simulink model "Master_Slave_Model_NOAZ"  (R2019b)
settings: Solver=VariableStepAuto  StartTime=0.0  StopTime=10  RelTol=1e-3
values from neighbouring files (symbols this model uses):
  Be = 5    [parameters.m]
  beta = 2*pi*Fc_h*Ts / (1+2*pi*Fc_h*Ts)    (= 0.0304590279514)    [parameters.m]
  Bh = 2*0.7*sqrt(Kh)    [parameters.m]
  delayCommM2S = 250    [parameters.m]
  delayCommS2M = 250    [parameters.m]
  dt = 0.01    [parameters.m]
  Fc_h = 5    [parameters.m]
  Fh_star = 25    [parameters.m]
  Jh = 0.002    [parameters.m]
  k_m = 19.34    [parameters.m]
  k_s = 19.34    [parameters.m]
  Kc2v_m = 2    [parameters.m]
  Kc2v_s = 2    [parameters.m]
  Kd_h = 0.5    [parameters.m]
  Kd_s = 0.5    [parameters.m]
  Ke = 10    [parameters.m]
  Kh = 25    [parameters.m]
  Kh_max = 50    [parameters.m]
  Kp_h = 1.2    [parameters.m]
  Kp_s = 1    [parameters.m]
  Kt2c_m = 1.182    [parameters.m]
  Kt2c_s = 1.182    [parameters.m]
  lArm_m = 0.1    [parameters.m]
  lArm_s = 0.1    [parameters.m]
  maxCurrent_m = 4.5    [parameters.m]
  maxCurrent_s = 4.5    [parameters.m]
  qe = 0.9    [parameters.m]
  stopTime = str2double(stopTime)    [parameters.m]
  tau_s = 1.217    [parameters.m]
  Ts = 0.001    [parameters.m]
  Variance = 0.0001    [parameters.m]
libraries: simulink_extras x16, dspsigops x16, dspsrcs4 x1
settings Model: Creator=Mirko  LastModifiedBy=Mirko

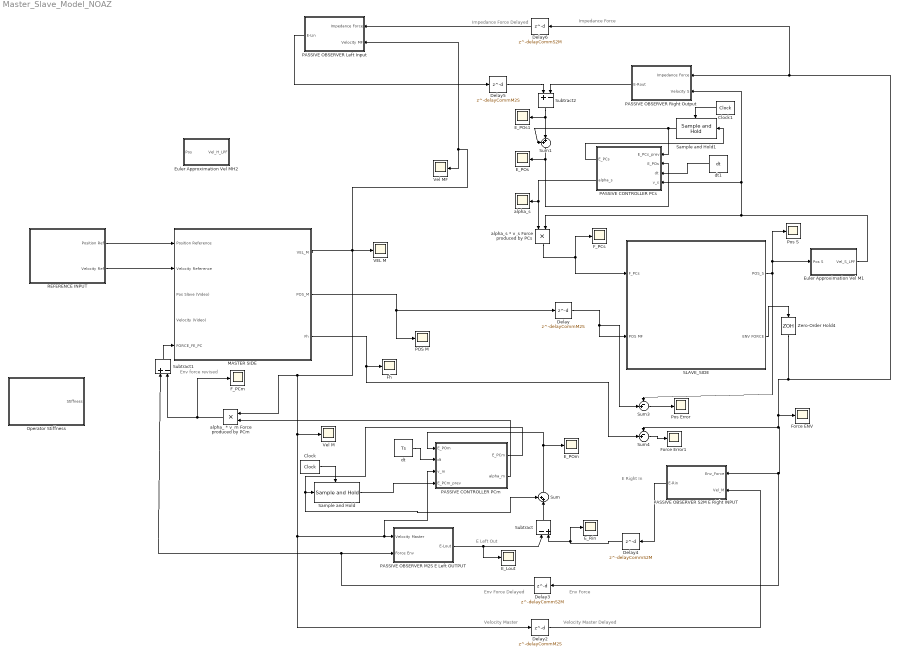
== system Master_Slave_Model_NOAZ ==
  note: Impedance Force Delayed
  note: Impedance Force
  note: Env force revised
  note: E Right In
  note: E Left Out
  note: Env Force Delayed
  note: Env Force
  note: Velocity Master
  note: Velocity Master Delayed
  Clock : simulink_extras/Flip Flops/Clock  period=Ts
  Clock1 : simulink_extras/Flip Flops/Clock  period=Ts
  Delay : Delay  DelayLength=delayCommM2S  InitialCondition=0  SampleTime=Ts
  Delay2 : Delay  DelayLength=delayCommM2S  InitialCondition=0  SampleTime=Ts
  Delay3 : Delay  DelayLength=delayCommS2M  InitialCondition=0  SampleTime=Ts
  Delay4 : Delay  DelayLength=delayCommS2M  InitialCondition=0
  Delay5 : Delay  DelayLength=delayCommM2S  InitialCondition=0  SampleTime=Ts
  Delay6 : Delay  DelayLength=delayCommS2M  InitialCondition=0  SampleTime=Ts
  E_Lout : Scope
  E_POm : Scope
  E_POs : Scope
  E_POs1 : Scope
  E_Rin : Scope
  Euler Approximation Vel M1 : Subsystem
  Euler Approximation Vel MH2 : Subsystem
  F_PCm : Scope
  F_PCs : Scope
  "Fh " : Scope
  Force ENV : Scope
  Force Error1 : Scope
  MASTER SIDE : Subsystem
  Operator Stiffness : Subsystem
  PASSIVE CONTROLLER PCm : MATLAB Function  TreatAsAtomicUnit=on
  PASSIVE CONTROLLER PCs : MATLAB Function  TreatAsAtomicUnit=on
  PASSIVE OBSERVER Left Input : Subsystem
  PASSIVE OBSERVER Right Output : Subsystem
  PASSIVE OBSERVER M2S E Left OUTPUT : Subsystem
  PASSIVE OBSERVER S2M E Right INPUT : Subsystem
  "POS M " : Scope
  Pos Error : Scope
  Pos S : Scope
  REFERENCE INPUT : Subsystem
  "SLAVE_SIDE " : Subsystem
  Sample and Hold : dspsigops/Sample and Hold  trig=Rising edge  initCond=0  latchinput=on
  Sample and Hold1 : dspsigops/Sample and Hold  trig=Rising edge  initCond=0  latchinput=on
  Subtract : Sum  Inputs=-|+
  Subtract1 : Sum  Inputs=+|-
  Subtract2 : Sum  Inputs=+|-
  Sum : Sum  Inputs=++|
  Sum1 : Sum  Inputs=++|
  Sum3 : Sum  Inputs=-+|
  Sum4 : Sum  Inputs=-+|
  VEL M : Scope
  "Vel M " : Scope
  Vel MF : Scope
  Zero-Order Hold4 : ZeroOrderHold  SampleTime=Ts
  alpha_ * v_m Force produced by PCm : Product
  alpha_s : Scope
  alpha_s * v_s Force produced by PCs : Product
  dt : Constant  Value=Ts
  dt1 : Constant  Value=dt
  wires:
  Delay3/1 -> PASSIVE OBSERVER M2S E Left OUTPUT/2(Force Env), Subtract1/1
  Delay2/1 -> PASSIVE OBSERVER S2M E Right INPUT/2("Vel_M ")
  PASSIVE OBSERVER M2S E Left OUTPUT/1(E-Lout) -> E_Lout/1, Subtract/1
  Subtract/1 -> Sum/2
  dt/1 -> PASSIVE CONTROLLER PCm/2(dt)
  PASSIVE CONTROLLER PCm/1(E_PCm) -> Sum/1, Sample and Hold/1
  Sum/1 -> E_POm/1, PASSIVE CONTROLLER PCm/1(E_POm)
  PASSIVE CONTROLLER PCm/2(alpha_m) -> alpha_ * v_m Force produced by PCm/2
  alpha_ * v_m Force produced by PCm/1 -> Subtract1/2, F_PCm/1
  Delay6/1 -> PASSIVE OBSERVER Left Input/1(Impedance Force)
  PASSIVE OBSERVER S2M E Right INPUT/1(E-Rin) -> Delay4/1
  Delay4/1 -> E_Rin/1, Subtract/2
  Euler Approximation Vel M1/1("Vel_S_LPF ") -> alpha_s * v_s Force produced by PCs/2, PASSIVE OBSERVER Right Output/2(Velocity S), PASSIVE CONTROLLER PCs/4(v_s)
  PASSIVE OBSERVER Left Input/1(E-Lin) -> Delay5/1
  Delay5/1 -> Subtract2/1
  PASSIVE OBSERVER Right Output/1(E-Rout) -> Subtract2/2
  dt1/1 -> PASSIVE CONTROLLER PCs/3(dt)
  Subtract2/1 -> E_POs1/1, Sum1/2
  PASSIVE CONTROLLER PCs/1(E_PCs) -> Sample and Hold1/1
  Sum1/1 -> E_POs/1, PASSIVE CONTROLLER PCs/2(E_POs)
  PASSIVE CONTROLLER PCs/2(alpha_s) -> alpha_s/1, alpha_s * v_s Force produced by PCs/1
  alpha_s * v_s Force produced by PCs/1 -> F_PCs/1, "SLAVE_SIDE "/1(F_PCs)
  Subtract1/1 -> MASTER SIDE/5("FORCE_FE_PC ")
  REFERENCE INPUT/1("Position Ref ") -> MASTER SIDE/1(Position Reference)
  Sum3/1 -> Pos Error/1
  Sum4/1 -> Force Error1/1
  MASTER SIDE/1(VEL_M) -> VEL M/1, PASSIVE OBSERVER Left Input/2(Velocity MF), Vel MF/1, alpha_ * v_m Force produced by PCm/1, "Vel M "/1, PASSIVE CONTROLLER PCm/3(v_m), PASSIVE OBSERVER M2S E Left OUTPUT/1(Velocity Master), Delay2/1
  Delay/1 -> Sum3/2, "SLAVE_SIDE "/2(POS MF)
  MASTER SIDE/3(Fh) -> Sum4/2, "Fh "/1
  "SLAVE_SIDE "/2(ENV FORCE) -> Zero-Order Hold4/1
  Zero-Order Hold4/1 -> Force ENV/1, PASSIVE OBSERVER S2M E Right INPUT/1(Env_Force), Delay3/1, Sum4/1, Delay6/1, PASSIVE OBSERVER Right Output/1(Impedance Force)
  MASTER SIDE/2(POS_M) -> "POS M "/1, Delay/1
  "SLAVE_SIDE "/1(POS_S) -> Euler Approximation Vel M1/1(Pos S), Pos S/1, Sum3/1
  Sample and Hold/1 -> PASSIVE CONTROLLER PCm/4(E_PCm_prev)
  Clock/1 -> Sample and Hold/Trigger
  Sample and Hold1/1 -> PASSIVE CONTROLLER PCs/1(E_PCs_prev), Sum1/1
  Clock1/1 -> Sample and Hold1/Trigger
  REFERENCE INPUT/2("Velocity Ref ") -> MASTER SIDE/2(Velocity Reference)

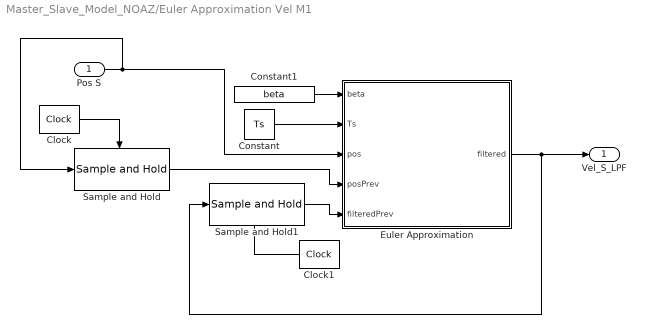
== system Master_Slave_Model_NOAZ/Euler Approximation Vel M1 ==
  Pos S : Inport
  Clock : simulink_extras/Flip Flops/Clock  period=Ts
  Clock1 : simulink_extras/Flip Flops/Clock  period=Ts
  Constant : Constant  Value=Ts
  Constant1 : Constant  Value=beta
  "Euler Approximation " : MATLAB Function  TreatAsAtomicUnit=on
  Sample and Hold : dspsigops/Sample and Hold  trig=Rising edge  initCond=0  latchinput=on
  Sample and Hold1 : dspsigops/Sample and Hold  trig=Rising edge  initCond=0  latchinput=on
  "Vel_S_LPF " : Outport
  wires:
  Pos S/1 -> Sample and Hold/1, "Euler Approximation "/3(pos)
  Constant/1 -> "Euler Approximation "/2(Ts)
  Sample and Hold/1 -> "Euler Approximation "/4(posPrev)
  Clock/1 -> Sample and Hold/Trigger
  Sample and Hold1/1 -> "Euler Approximation "/5(filteredPrev)
  "Euler Approximation "/1(filtered) -> "Vel_S_LPF "/1, Sample and Hold1/1
  Clock1/1 -> Sample and Hold1/Trigger
  Constant1/1 -> "Euler Approximation "/1(beta)

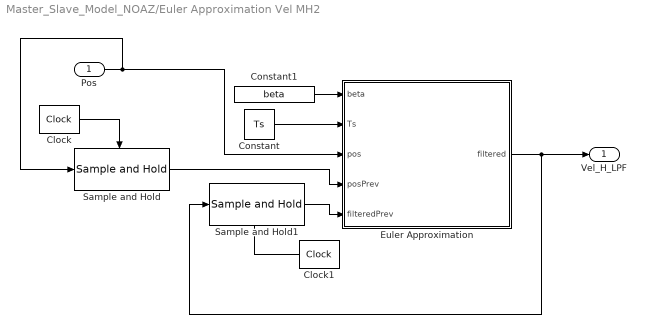
== system Master_Slave_Model_NOAZ/Euler Approximation Vel MH2 ==
  Pos : Inport
  Clock : simulink_extras/Flip Flops/Clock  period=Ts
  Clock1 : simulink_extras/Flip Flops/Clock  period=Ts
  Constant : Constant  Value=Ts
  Constant1 : Constant  Value=beta
  "Euler Approximation " : MATLAB Function  TreatAsAtomicUnit=on
  Sample and Hold : dspsigops/Sample and Hold  trig=Rising edge  initCond=0  latchinput=on
  Sample and Hold1 : dspsigops/Sample and Hold  trig=Rising edge  initCond=0  latchinput=on
  "Vel_H_LPF " : Outport
  wires:
  Pos/1 -> Sample and Hold/1, "Euler Approximation "/3(pos)
  Constant/1 -> "Euler Approximation "/2(Ts)
  Sample and Hold/1 -> "Euler Approximation "/4(posPrev)
  Clock/1 -> Sample and Hold/Trigger
  Sample and Hold1/1 -> "Euler Approximation "/5(filteredPrev)
  "Euler Approximation "/1(filtered) -> "Vel_H_LPF "/1, Sample and Hold1/1
  Clock1/1 -> Sample and Hold1/Trigger
  Constant1/1 -> "Euler Approximation "/1(beta)

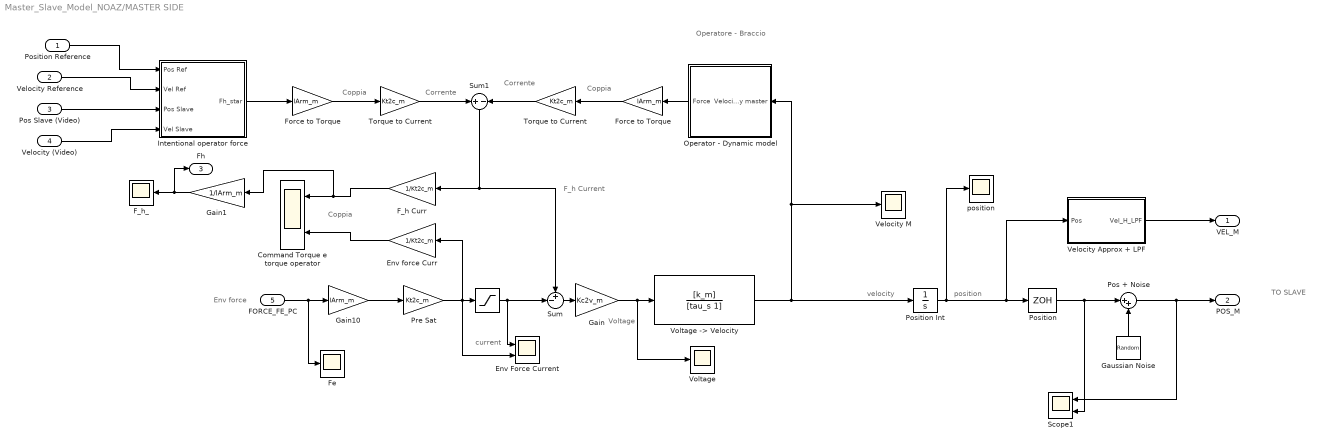
== system Master_Slave_Model_NOAZ/MASTER SIDE ==
  note: Env force
  note: F_h Current
  note: Coppia
  note: Corrente
  note: Coppia
  note: Corrente
  note: Coppia
  note: Operatore - Braccio
  note: current
  note: Voltage
  note: position
  note: velocity
  note: TO SLAVE
  Position Reference : Inport
  Velocity Reference : Inport  Port=2
  Pos Slave (Video) : Inport  Port=3
  Velocity (Video) : Inport  Port=4
  "FORCE_FE_PC " : Inport  Port=5
  " " : Saturate  UpperLimit=maxCurrent_m  LowerLimit=-maxCurrent_m
  "Command Torque e torque operator " : Scope  NumInputPorts=2
  Env Force Current : Scope  NumInputPorts=2
  Env force Curr : Gain  Gain=1/Kt2c_m
  F_h Curr : Gain  Gain=1/Kt2c_m
  "F_h_ " : Scope
  Fe : Scope
  Force to Torque : Gain  Gain=lArm_m
  "Force to Torque " : Gain  Gain=lArm_m
  Gain : Gain  Gain=Kc2v_m
  Gain1 : Gain  Gain=1/lArm_m
  Gain10 : Gain  Gain=lArm_m
  "Gaussian Noise " : RandomNumber  Variance=Variance  SampleTime=Ts
  Intentional operator force : Subsystem
  Operator - Dynamic model : Subsystem
  Pos + Noise : Sum  Inputs=|++
  Position : ZeroOrderHold  SampleTime=Ts
  "Position Int " : Integrator
  Pre Sat : Gain  Gain=Kt2c_m
  Scope1 : Scope  NumInputPorts=2
  Sum : Sum  Inputs=+-|
  Sum1 : Sum  Inputs=+-
  Torque to Current : Gain  Gain=Kt2c_m
  "Torque to Current " : Gain  Gain=Kt2c_m
  "Velocity Approx + LPF " : Subsystem
  Velocity M : Scope
  Voltage : Scope
  "Voltage -> Velocity" : TransferFcn  Numerator=[k_m]  Denominator=[tau_s 1]
  position : Scope
  VEL_M : Outport
  POS_M : Outport  Port=2
  Fh : Outport  Port=3
  wires:
  Pre Sat/1 -> Env Force Current/2, Env force Curr/1, " "/1
  "Position Int "/1 -> "Velocity Approx + LPF "/1(Pos), Position/1, position/1
  "Voltage -> Velocity"/1 -> Velocity M/1, Operator - Dynamic model/1("Velocity master "), "Position Int "/1
  Sum1/1 -> Sum/1, F_h Curr/1
  "Force to Torque "/1 -> Torque to Current/1
  F_h Curr/1 -> Gain1/1, "Command Torque e torque operator "/1
  Force to Torque/1 -> "Torque to Current "/1
  "Torque to Current "/1 -> Sum1/2
  Env force Curr/1 -> "Command Torque e torque operator "/2
  Torque to Current/1 -> Sum1/1
  Position Reference/1 -> Intentional operator force/1(Pos Ref)
  Gain/1 -> Voltage/1, "Voltage -> Velocity"/1
  Sum/1 -> Gain/1
  "FORCE_FE_PC "/1 -> Fe/1, Gain10/1
  Gain10/1 -> Pre Sat/1
  Operator - Dynamic model/1(Force) -> Force to Torque/1
  " "/1 -> Sum/2, Env Force Current/1
  Gain1/1 -> Fh/1, "F_h_ "/1
  "Gaussian Noise "/1 -> Pos + Noise/2
  Pos + Noise/1 -> Scope1/1, POS_M/1
  Position/1 -> Scope1/2, Pos + Noise/1
  "Velocity Approx + LPF "/1("Vel_H_LPF ") -> VEL_M/1
  Velocity Reference/1 -> Intentional operator force/2(Vel Ref)
  Intentional operator force/1("Fh_star ") -> "Force to Torque "/1
  Pos Slave (Video)/1 -> Intentional operator force/3(Pos Slave)
  Velocity (Video)/1 -> Intentional operator force/4(Vel Slave)

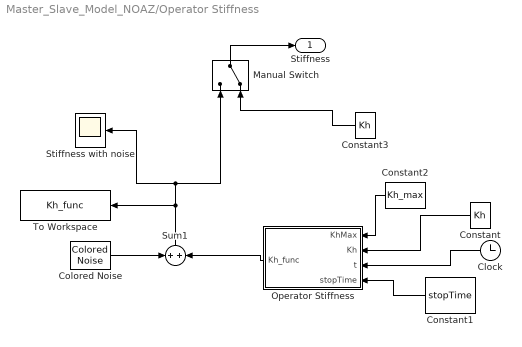
== system Master_Slave_Model_NOAZ/Operator Stiffness ==
  Clock : Clock
  Colored Noise : dspsrcs4/Colored Noise  Color=white  InverseFrequencyPower=1  BoundedOutput=off  NumChannels=1  OutputDataType=double  SamplesPerFrame=1  SampleTime=0.01  RandomStream=mt19937ar with seed  Seed=67  SimulateUsing=Interpreted execution
      settings: SourceProductName=DSP System Toolbox  SourceProductBaseCode=DS
  Constant : Constant  Value=Kh
  Constant1 : Constant  Value=stopTime
  Constant2 : Constant  Value=Kh_max
  Constant3 : Constant  Value=Kh
  Manual Switch : ManualSwitch  CurrentSetting=0
  "Operator Stiffness " : MATLAB Function  TreatAsAtomicUnit=on
  Stiffness with noise : Scope
  Sum1 : Sum
  To Workspace : ToWorkspace  VariableName=Kh_func  SaveFormat=Structure With Time  SampleTime=-1
      settings: Save2DSignal=2-D array (concatenate along first dimension)
  Stiffness : Outport
  wires:
  Constant3/1 -> Manual Switch/2
  Sum1/1 -> To Workspace/1, Manual Switch/1, Stiffness with noise/1
  Constant2/1 -> "Operator Stiffness "/1(KhMax)
  "Operator Stiffness "/1(Kh_func) -> Sum1/2
  Clock/1 -> "Operator Stiffness "/3(t)
  Colored Noise/1 -> Sum1/1
  Constant/1 -> "Operator Stiffness "/2(Kh)
  Constant1/1 -> "Operator Stiffness "/4(stopTime)
  Manual Switch/1 -> Stiffness/1

== system Master_Slave_Model_NOAZ/PASSIVE OBSERVER Left Input ==
  Impedance Force : Inport
  Velocity MF : Inport  Port=2
  Add : Sum
  Clock : simulink_extras/Flip Flops/Clock  period=Ts
  Product : Product
  Sample and Hold : dspsigops/Sample and Hold  trig=Rising edge  initCond=0  latchinput=on
  E-Lin : Outport
  wires:
  Velocity MF/1 -> Product/1
  Impedance Force/1 -> Product/2
  Product/1 -> Add/2
  Sample and Hold/1 -> Add/1
  Add/1 -> Sample and Hold/1, E-Lin/1
  Clock/1 -> Sample and Hold/Trigger

== system Master_Slave_Model_NOAZ/PASSIVE OBSERVER Right Output ==
  Impedance Force : Inport
  Velocity S : Inport  Port=2
  Add : Sum
  Clock : simulink_extras/Flip Flops/Clock  period=Ts
  Product : Product
  Sample and Hold : dspsigops/Sample and Hold  trig=Rising edge  initCond=0  latchinput=on
  E-Rout : Outport
  wires:
  Velocity S/1 -> Product/1
  Impedance Force/1 -> Product/2
  Product/1 -> Add/2
  Sample and Hold/1 -> Add/1
  Add/1 -> Sample and Hold/1, E-Rout/1
  Clock/1 -> Sample and Hold/Trigger

== system Master_Slave_Model_NOAZ/PASSIVE OBSERVER M2S E Left OUTPUT ==
  Velocity Master : Inport
  Force Env : Inport  Port=2
  Add : Sum
  Clock : simulink_extras/Flip Flops/Clock  period=Ts
  Product : Product
  Sample and Hold : dspsigops/Sample and Hold  trig=Rising edge  initCond=0  latchinput=on
  E-Lout : Outport
  wires:
  Velocity Master/1 -> Product/1
  Force Env/1 -> Product/2
  Product/1 -> Add/2
  Sample and Hold/1 -> Add/1
  Add/1 -> Sample and Hold/1, E-Lout/1
  Clock/1 -> Sample and Hold/Trigger

== system Master_Slave_Model_NOAZ/PASSIVE OBSERVER S2M E Right INPUT ==
  Env_Force : Inport
  "Vel_M " : Inport  Port=2
  Add : Sum
  Clock : simulink_extras/Flip Flops/Clock  period=Ts
  Product : Product
  Sample and Hold : dspsigops/Sample and Hold  trig=Rising edge  initCond=0  latchinput=on
  E-Rin : Outport
  wires:
  Env_Force/1 -> Product/1
  "Vel_M "/1 -> Product/2
  Product/1 -> Add/2
  Add/1 -> Sample and Hold/1, E-Rin/1
  Sample and Hold/1 -> Add/1
  Clock/1 -> Sample and Hold/Trigger

== system Master_Slave_Model_NOAZ/REFERENCE INPUT ==
  Derivative : Derivative
  Manual Switch : ManualSwitch  CurrentSetting=0
  Sine Wave : Sin  Amplitude=Fh_star  SampleTime=0
  Step : Step  After=Fh_star  SampleTime=0
  Transfer Fcn : TransferFcn  Numerator=[2*pi*Fc_h]  Denominator=[1 2*pi*Fc_h]
  "Position Ref " : Outport
  "Velocity Ref " : Outport  Port=2
  wires:
  Sine Wave/1 -> Manual Switch/1
  Step/1 -> Transfer Fcn/1
  Transfer Fcn/1 -> Manual Switch/2
  Manual Switch/1 -> Derivative/1, "Position Ref "/1
  Derivative/1 -> "Velocity Ref "/1

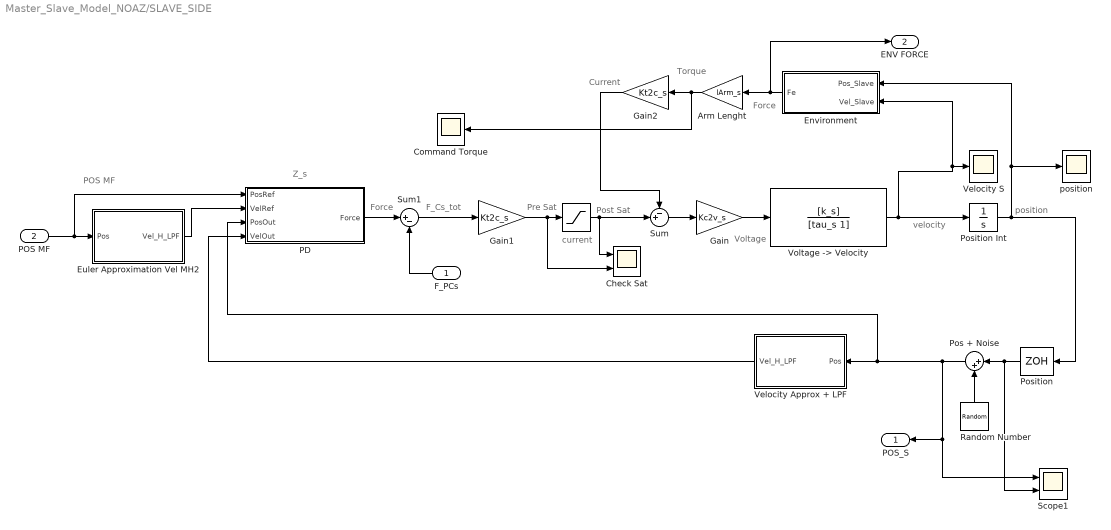
== system Master_Slave_Model_NOAZ/SLAVE_SIDE  ==
  note: Post Sat
  note: Pre Sat
  note: POS MF
  note: current
  note: Force
  note: velocity
  note: position
  note: Current
  note: Voltage
  note: Torque
  note: Z_s
  note: Force
  note: F_Cs_tot
  F_PCs : Inport
  POS MF : Inport  Port=2
  " " : Saturate  UpperLimit=maxCurrent_s  LowerLimit=-maxCurrent_s
  Arm Lenght : Gain  Gain=lArm_s
  Check Sat : Scope  NumInputPorts=2
  Command Torque : Scope
  "Environment " : Subsystem
  Euler Approximation Vel MH2 : Subsystem
  Gain : Gain  Gain=Kc2v_s
  Gain1 : Gain  Gain=Kt2c_s
  Gain2 : Gain  Gain=Kt2c_s
  PD : Subsystem
  Pos + Noise : Sum  Inputs=|++
  Position : ZeroOrderHold  SampleTime=Ts
  Position Int : Integrator
  Random Number : RandomNumber  Variance=Variance  SampleTime=Ts
  Scope1 : Scope  NumInputPorts=2
  Sum : Sum  Inputs=-+|
  Sum1 : Sum  Inputs=|+-
  "Velocity Approx + LPF " : Subsystem
  Velocity S : Scope
  "Voltage -> Velocity " : TransferFcn  Numerator=[k_s]  Denominator=[tau_s 1]
  position : Scope
  POS_S : Outport
  ENV FORCE : Outport  Port=2
  wires:
  PD/1(Force) -> Sum1/1
  Gain1/1 -> Check Sat/2, " "/1
  Gain2/1 -> Sum/1
  "Environment "/1(Fe) -> ENV FORCE/1, Arm Lenght/1
  "Voltage -> Velocity "/1 -> Position Int/1, Velocity S/1, "Environment "/2("Vel_Slave ")
  Sum/1 -> Gain/1
  Gain/1 -> "Voltage -> Velocity "/1
  Sum1/1 -> Gain1/1
  " "/1 -> Check Sat/1, Sum/2
  Arm Lenght/1 -> Command Torque/1, Gain2/1
  F_PCs/1 -> Sum1/2
  Euler Approximation Vel MH2/1("Vel_H_LPF ") -> PD/2(VelRef)
  POS MF/1 -> PD/1(PosRef), Euler Approximation Vel MH2/1(Pos)
  Random Number/1 -> Pos + Noise/2
  Pos + Noise/1 -> PD/3(PosOut), "Velocity Approx + LPF "/1(Pos), POS_S/1, Scope1/1
  Position/1 -> Scope1/2, Pos + Noise/1
  Position Int/1 -> Position/1, position/1, "Environment "/1(Pos_Slave)
  "Velocity Approx + LPF "/1("Vel_H_LPF ") -> PD/4(VelOut)

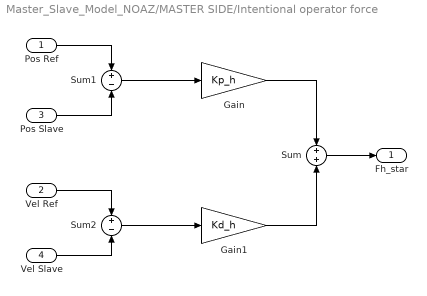
== system Master_Slave_Model_NOAZ/MASTER SIDE/Intentional operator force ==
  Pos Ref : Inport
  Vel Ref : Inport  Port=2
  Pos Slave : Inport  Port=3
  Vel Slave : Inport  Port=4
  Gain : Gain  Gain=Kp_h
  Gain1 : Gain  Gain=Kd_h
  Sum : Sum
  Sum1 : Sum  Inputs=+-
  Sum2 : Sum  Inputs=+-
  "Fh_star " : Outport
  wires:
  Sum/1 -> "Fh_star "/1
  Pos Ref/1 -> Sum1/1
  Pos Slave/1 -> Sum1/2
  Vel Ref/1 -> Sum2/1
  Vel Slave/1 -> Sum2/2
  Sum1/1 -> Gain/1
  Sum2/1 -> Gain1/1
  Gain1/1 -> Sum/2
  Gain/1 -> Sum/1

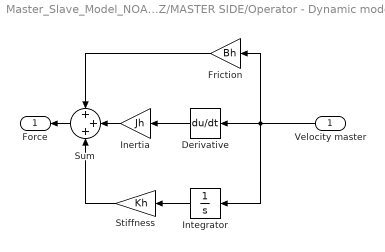
== system Master_Slave_Model_NOAZ/MASTER SIDE/Operator - Dynamic model ==
  "Velocity master " : Inport
  Derivative : Derivative  CoefficientInTFapproximation=0.01
  Friction : Gain  Gain=Bh
  Inertia : Gain  Gain=Jh
  Integrator : Integrator
  "Stiffness " : Gain  Gain=Kh
  Sum : Sum  Inputs=+++
  Force : Outport
  wires:
  "Velocity master "/1 -> Friction/1, Integrator/1, Derivative/1
  Derivative/1 -> Inertia/1
  Inertia/1 -> Sum/2
  Friction/1 -> Sum/1
  Sum/1 -> Force/1
  Integrator/1 -> "Stiffness "/1
  "Stiffness "/1 -> Sum/3

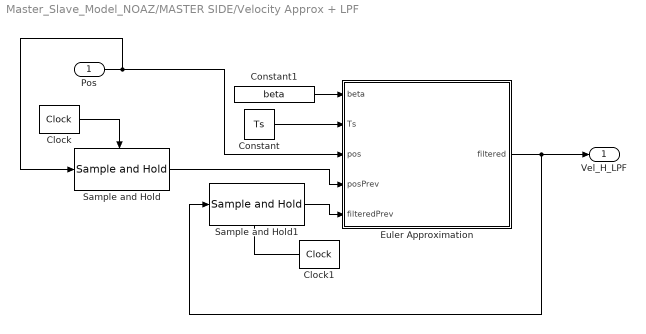
== system Master_Slave_Model_NOAZ/MASTER SIDE/Velocity Approx + LPF  ==
  Pos : Inport
  Clock : simulink_extras/Flip Flops/Clock  period=Ts
  Clock1 : simulink_extras/Flip Flops/Clock  period=Ts
  Constant : Constant  Value=Ts
  Constant1 : Constant  Value=beta
  "Euler Approximation " : MATLAB Function  TreatAsAtomicUnit=on
  Sample and Hold : dspsigops/Sample and Hold  trig=Rising edge  initCond=0  latchinput=on
  Sample and Hold1 : dspsigops/Sample and Hold  trig=Rising edge  initCond=0  latchinput=on
  "Vel_H_LPF " : Outport
  wires:
  Pos/1 -> Sample and Hold/1, "Euler Approximation "/3(pos)
  Constant/1 -> "Euler Approximation "/2(Ts)
  Sample and Hold/1 -> "Euler Approximation "/4(posPrev)
  Clock/1 -> Sample and Hold/Trigger
  Sample and Hold1/1 -> "Euler Approximation "/5(filteredPrev)
  "Euler Approximation "/1(filtered) -> "Vel_H_LPF "/1, Sample and Hold1/1
  Clock1/1 -> Sample and Hold1/Trigger
  Constant1/1 -> "Euler Approximation "/1(beta)

== system Master_Slave_Model_NOAZ/SLAVE_SIDE /Environment  ==
  Pos_Slave : Inport
  "Vel_Slave " : Inport  Port=2
  Environment Behaviour : MATLAB Function  TreatAsAtomicUnit=on
  Environment Position : Constant  Value=qe
  Stiffness : Constant  Value=Ke
  Viscous Friction : Constant  Value=Be
  Fe : Outport
  wires:
  Pos_Slave/1 -> Environment Behaviour/1(x_s)
  "Vel_Slave "/1 -> Environment Behaviour/2(dot_x_s)
  Environment Position/1 -> Environment Behaviour/3(qe)
  Viscous Friction/1 -> Environment Behaviour/4(Be)
  Stiffness/1 -> Environment Behaviour/5(Ke)
  Environment Behaviour/1(Fe) -> Fe/1

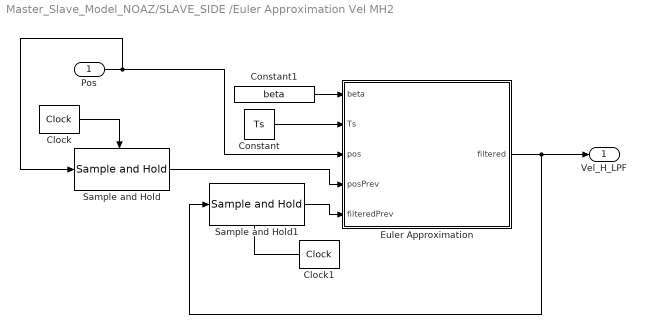
== system Master_Slave_Model_NOAZ/SLAVE_SIDE /Euler Approximation Vel MH2 ==
  Pos : Inport
  Clock : simulink_extras/Flip Flops/Clock  period=Ts
  Clock1 : simulink_extras/Flip Flops/Clock  period=Ts
  Constant : Constant  Value=Ts
  Constant1 : Constant  Value=beta
  "Euler Approximation " : MATLAB Function  TreatAsAtomicUnit=on
  Sample and Hold : dspsigops/Sample and Hold  trig=Rising edge  initCond=0  latchinput=on
  Sample and Hold1 : dspsigops/Sample and Hold  trig=Rising edge  initCond=0  latchinput=on
  "Vel_H_LPF " : Outport
  wires:
  Pos/1 -> Sample and Hold/1, "Euler Approximation "/3(pos)
  Constant/1 -> "Euler Approximation "/2(Ts)
  Sample and Hold/1 -> "Euler Approximation "/4(posPrev)
  Clock/1 -> Sample and Hold/Trigger
  Sample and Hold1/1 -> "Euler Approximation "/5(filteredPrev)
  "Euler Approximation "/1(filtered) -> "Vel_H_LPF "/1, Sample and Hold1/1
  Clock1/1 -> Sample and Hold1/Trigger
  Constant1/1 -> "Euler Approximation "/1(beta)

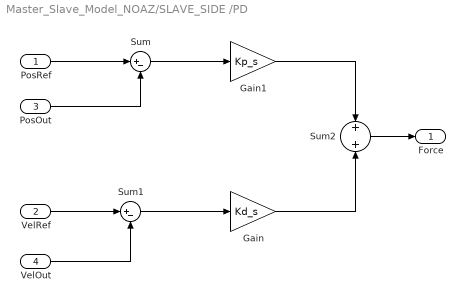
== system Master_Slave_Model_NOAZ/SLAVE_SIDE /PD ==
  PosRef : Inport
  VelRef : Inport  Port=2
  PosOut : Inport  Port=3
  VelOut : Inport  Port=4
  Gain : Gain  Gain=Kd_s
  Gain1 : Gain  Gain=Kp_s
  Sum : Sum  Inputs=|+-
  Sum1 : Sum  Inputs=|+-
  Sum2 : Sum
  Force : Outport
  wires:
  PosRef/1 -> Sum/1
  PosOut/1 -> Sum/2
  VelRef/1 -> Sum1/1
  VelOut/1 -> Sum1/2
  Sum1/1 -> Gain/1
  Sum/1 -> Gain1/1
  Gain1/1 -> Sum2/1
  Gain/1 -> Sum2/2
  Sum2/1 -> Force/1

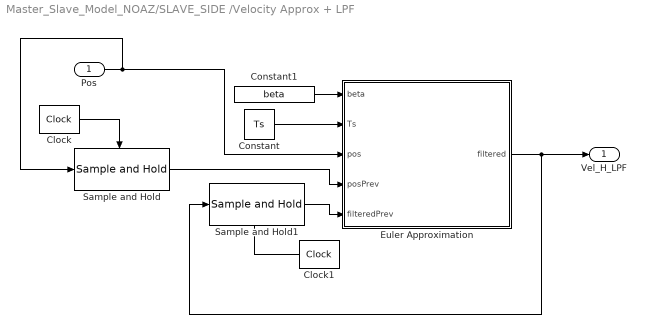
== system Master_Slave_Model_NOAZ/SLAVE_SIDE /Velocity Approx + LPF  ==
  Pos : Inport
  Clock : simulink_extras/Flip Flops/Clock  period=Ts
  Clock1 : simulink_extras/Flip Flops/Clock  period=Ts
  Constant : Constant  Value=Ts
  Constant1 : Constant  Value=beta
  "Euler Approximation " : MATLAB Function  TreatAsAtomicUnit=on
  Sample and Hold : dspsigops/Sample and Hold  trig=Rising edge  initCond=0  latchinput=on
  Sample and Hold1 : dspsigops/Sample and Hold  trig=Rising edge  initCond=0  latchinput=on
  "Vel_H_LPF " : Outport
  wires:
  Pos/1 -> Sample and Hold/1, "Euler Approximation "/3(pos)
  Constant/1 -> "Euler Approximation "/2(Ts)
  Sample and Hold/1 -> "Euler Approximation "/4(posPrev)
  Clock/1 -> Sample and Hold/Trigger
  Sample and Hold1/1 -> "Euler Approximation "/5(filteredPrev)
  "Euler Approximation "/1(filtered) -> "Vel_H_LPF "/1, Sample and Hold1/1
  Clock1/1 -> Sample and Hold1/Trigger
  Constant1/1 -> "Euler Approximation "/1(beta)

== matlab function Master_Slave_Model_NOAZ/PASSIVE CONTROLLER PCm ==
  data: E_POm input; E_PCm output; dt input; v_m input; E_PCm_prev input; alpha_m output
function [E_PCm, alpha_m]= PC_m(E_POm, dt, v_m, E_PCm_prev)

if (E_POm < 0 && v_m ~= 0)
    alpha_m = (-E_POm)/dt*v_m^2;
else
    alpha_m = 0;
end

E_PCm = E_PCm_prev + (alpha_m*v_m^2)*dt;

== matlab function Master_Slave_Model_NOAZ/SLAVE_SIDE /Environment /Environment Behaviour ==
  data: x_s input; Fe output; dot_x_s input; qe input; Be input; Ke input
function Fe = Env(x_s, dot_x_s, qe, Be, Ke)
    
    if(x_s > qe)
        Fe = Ke*(x_s - qe) + Be*dot_x_s;
    else
        Fe = 0;
    end

== matlab function Master_Slave_Model_NOAZ/PASSIVE CONTROLLER PCs ==
  data: E_PCs_prev input; E_POs input; E_PCs output; dt input; v_s input; alpha_s output
function [E_PCs, alpha_s]= PC_s(E_PCs_prev, E_POs, dt, v_s)

if (E_POs < 0 && v_s ~= 0)
    alpha_s = (-E_POs)/dt*v_s^2;
else
    alpha_s = 0;
end

E_PCs = E_PCs_prev + (alpha_s*v_s^2)*dt;

== matlab function Master_Slave_Model_NOAZ/Operator Stiffness/Operator Stiffness  ==
  data: KhMax input; Kh input; Kh_func output; t input; stopTime input
function Kh_func = stiffness(KhMax, Kh, t, stopTime)
%Solving cubic polynomial function to model the operator stiffness
%(f'(begin) + f'(end) - 2*f(begin))(x/k)^3 + (3*f(end) - 2*f'(begin) - f'(end))(x/k)^2 + f'(begin)x/k + f(begin)

begin = 0.5;

endTime = stopTime-1;

df_begin = 0;
df_end = 0;
f_end = KhMax - Kh;

if t < begin
    Kh_func = Kh;
else
    Kh_func = (df_begin + df_end - 2*f_end)*((t-begin)/endTime)^3 + (3*f_end - 2*df_begin - df_end)*((t-begin)/endTime)^2 + (df_begin)*((t-begin)/endTime) + Kh;
end

== matlab function Master_Slave_Model_NOAZ/Euler Approximation Vel MH2/Euler Approximation  ==
  data: beta input; Ts input; filtered output; pos input; posPrev input; filteredPrev input
function filtered = EulApprox(beta, Ts, pos, posPrev, filteredPrev)

eul= (pos - posPrev)/Ts;
filtered = beta*eul + (1-beta)*filteredPrev;

== matlab function Master_Slave_Model_NOAZ/SLAVE_SIDE /Euler Approximation Vel MH2/Euler Approximation  ==
  data: beta input; Ts input; filtered output; pos input; posPrev input; filteredPrev input
function filtered = EulApprox(beta, Ts, pos, posPrev, filteredPrev)

eul= (pos - posPrev)/Ts;
filtered = beta*eul + (1-beta)*filteredPrev;

== matlab function Master_Slave_Model_NOAZ/SLAVE_SIDE /Velocity Approx + LPF /Euler Approximation  ==
  data: beta input; Ts input; filtered output; pos input; posPrev input; filteredPrev input
function filtered = EulApprox(beta, Ts, pos, posPrev, filteredPrev)

eul= (pos - posPrev)/Ts;
filtered = beta*eul + (1-beta)*filteredPrev;

== matlab function Master_Slave_Model_NOAZ/Euler Approximation Vel M1/Euler Approximation  ==
  data: beta input; Ts input; filtered output; pos input; posPrev input; filteredPrev input
function filtered = EulApprox(beta, Ts, pos, posPrev, filteredPrev)

eul= (pos - posPrev)/Ts;
filtered = beta*eul + (1-beta)*filteredPrev;

== matlab function Master_Slave_Model_NOAZ/MASTER SIDE/Velocity Approx + LPF /Euler Approximation  ==
  data: beta input; Ts input; filtered output; pos input; posPrev input; filteredPrev input
function filtered = EulApprox(beta, Ts, pos, posPrev, filteredPrev)

eul= (pos - posPrev)/Ts;
filtered = beta*eul + (1-beta)*filteredPrev;
